simulink model "Lab2_Simulink_Design_Part3_3"  (R2020a)
settings: Solver=VariableStepAuto  StartTime=0.0  StopTime=10.0  RelTol=1e-3
settings Model: Creator=mati1  LastModifiedBy=mati1

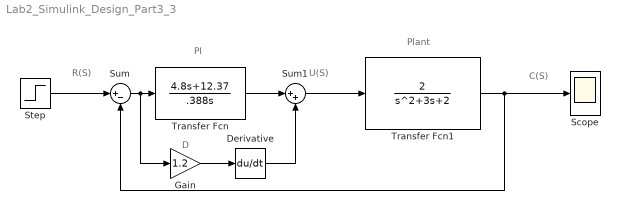
== system Lab2_Simulink_Design_Part3_3 ==
  note: D
  note: PI
  note: R(S)
  note: C(S)
  note: U(S)
  note: Plant
  Derivative : Derivative
  Gain : Gain  Gain=1.2
  Scope : Scope
  Step : Step  Before=1  SampleTime=0
  Sum : Sum  Inputs=|+-
  Sum1 : Sum  Inputs=|++
  Transfer Fcn : TransferFcn  Numerator=[4.8 12.37]  Denominator=[.388 0]
  Transfer Fcn1 : TransferFcn  Numerator=[2]  Denominator=[1 3 2]
  wires:
  Step/1 -> Sum/1
  Transfer Fcn1/1 -> Sum/2, Scope/1
  Sum/1 -> Gain/1, Transfer Fcn/1
  Sum1/1 -> Transfer Fcn1/1
  Transfer Fcn/1 -> Sum1/1
  Gain/1 -> Derivative/1
  Derivative/1 -> Sum1/2
